simulink model "Controller"  (R2021a)
settings: Solver=VariableStepAuto  StartTime=0.0  StopTime=10.0  RelTol=1e-3
settings Model: DataDictionary=Thermostat.sldd  Creator=smrh1  LastModifiedBy=smrh1

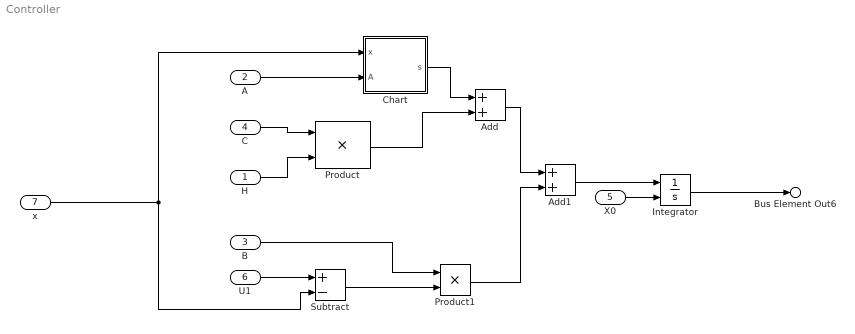
== system Controller ==
  H : Inport
  A : Inport  Port=2
  B : Inport  Port=3
  C : Inport  Port=4
  X0 : Inport  Port=5
  U1 : Inport  Port=6
  x : Inport  Port=7
  Add : Sum
  Add1 : Sum
  Chart : Stateflow chart  TreatAsAtomicUnit=on
  Integrator : Integrator  InitialConditionSource=external
  Product : Product
  Product1 : Product
  Subtract : Sum  Inputs=+-
  Bus Element Out6 : Outport  PortName=X
  wires:
  Integrator/1 -> Bus Element Out6/1
  H/1 -> Product/2
  Product1/1 -> Add1/2
  Chart/1(s) -> Add/1
  x/1 -> Subtract/2, Chart/1(x)
  Product/1 -> Add/2
  B/1 -> Product1/1
  Subtract/1 -> Product1/2
  Add1/1 -> Integrator/1
  X0/1 -> Integrator/2
  C/1 -> Product/1
  Add/1 -> Add1/1
  U1/1 -> Subtract/1
  A/1 -> Chart/2(A)

== stateflow chart Controller/Chart ==
  state s3
    du:
    s(1) = A(1,2)*(x(2)-x(1)) + A(1,3)*(x(3)-x(1)) + A(1,4)*(x(4)-x(1));
    s(2) = A(2,1)*(x(1)-x(2)) + A(2,3)*(x(3)-x(2)) + A(2,4)*(x(4)-x(2));
    s(3) = A(3,1)*(x(1)-x(3)) + A(3,2)*(x(2)-x(3)) + A(3,4)*(x(4)-x(3));
    s(4) = A(4,1)*(x(1)-x(4)) + A(4,2)*(x(2)-x(4)) + A(4,3)*(x(3)-x(4));
  (default) -> s3 : {s=[0,0,0,0];}
  data: x input; A input; s output
